simulink model "sgMdl_IO324_AnalogLoopbackDMA"  (R2024b)
settings: Solver=FixedStepAuto  StartTime=0.0  StopTime=inf  RelTol=1e-3
undefined symbols (not defined in the file): Ended, IO3xx, Pull, pull, Single, up
libraries: slrealtimeloglib x7, speedgoatlib_fpga_analog_io x3, speedgoatlib_interrupt x2, speedgoatlib_fpga x1
Description:
  | IO324 - Analog Loopback with DMA and Frame-Based Processing
settings Model: ModifiedByFormat=Speedgoat  SimulationMode=external  ExtModeTrigDuration=100000  Creator=Speedgoat  LastModifiedBy=Speedgoat
settings SolverCC: ConcurrentTasks=on  PositivePriorityOrder=on
settings DataIOCC: SaveFormat=StructureWithTime
settings OptimizationCC: BlockReduction=off  OptimizeBlockIOStorage=off  BufferReuse=off  ReuseModelBlockBuffer=off
settings DebuggingCC: UnderspecifiedInitializationDetection=Classic  MergeDetectMultiDrivingBlocksExec=none  TasksWithSamePriorityMsg=none
settings HardwareCC: ProdBitPerLong=64  ProdLongLongMode=on  ProdHWDeviceType=Intel->x86-64 (Linux 64)
settings ModelReferenceCC: EnableRefExpFcnMdlSchedulingChecks=on  PropagateSignalLabelsOutOfModel=off
settings RTWCC: Description=Speedgoat Real-Time Target Machine  SystemTargetFile=speedgoat.tlc  TemplateMakefile=slrealtime_default_tmf  PostCodeGenCommand=sg.model.build.makeCfg(bdroot, buildInfo);  Toolchain=Simulink Real-Time Toolchain  BuildConfiguration=Faster Runs  TargetLang=C++  GPUComputeCapability=3.5
settings SimulinkRealTimeTargetCC: SubcomponentCodeInterfacePackaging=Reusable function  InstructionSetFMA=off  LogToMDFFile=off  SLRTForcePollingMode=on  SLRTFileLogMaxRuns=10
settings ConfigComp: CovBoundaryAbsTol=1.0e-5

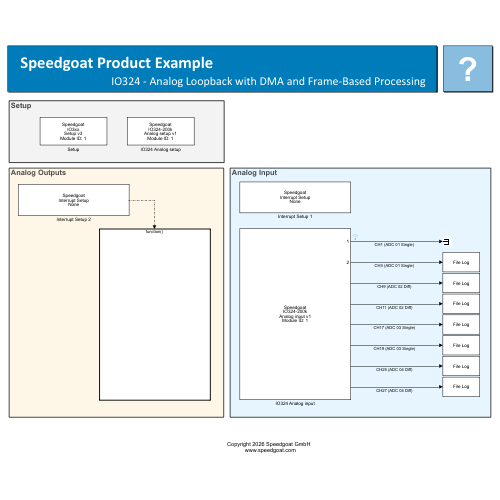
[thumbnail: Simulink's stored preview of the top-level diagram]
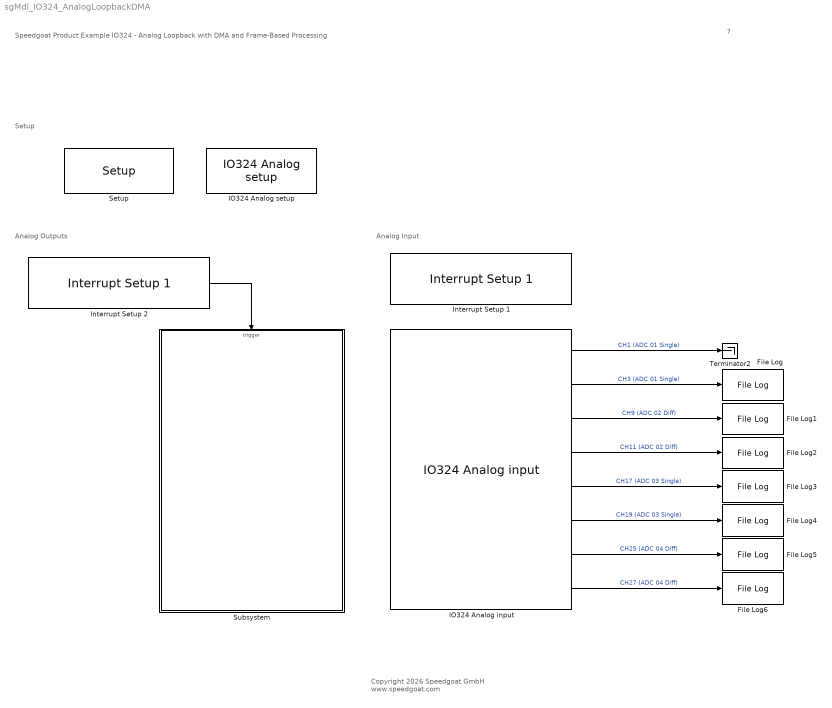
== system sgMdl_IO324_AnalogLoopbackDMA ==
  note: Analog Outputs
  note: Analog Input
  note: Setup
  note: Speedgoat Product Example
      | IO324 - Analog Loopback with DMA and Frame-Based Processing
  note: ?
  note: Copyright 2026 Speedgoat GmbH
      |  www.speedgoat.com
  File Log{,1..6} (7 alike) : slrealtimeloglib/File Log  decimation=1  inputProcessing=Elements as channels (sample based)
  IO324 Analog input : speedgoatlib_fpga_analog_io/IO324/IO324 Analog input  Priority=1  id=1  parSampleTime=-1  parPciSlot=-1  parAiChannels=[1 3 9 11 17 19 25 27]  parAiTriggerMode=[2 2 2 2]  parAiReadPrevValue=0  parAiEnableFrame=1  parAiVoltageRange=[2 2 2 2 2 2 2 2]  parAdcCoupling=[1 1 1 1]  parAdcContSampling=0  parAdcDmaEnable=0  parAdcActiveDmaDevices=[1 1 1 1]  parAiFrameSize=100
      settings: SourceProductName=Simulink Real-Time: Speedgoat I/O Blockset
  IO324 Analog setup : speedgoatlib_fpga_analog_io/IO324/IO324 Analog setup  id=1  parEnableCodeModule1=off  parEnableCodeModule2=off  parEnableCodeModule3=off  parEnableCodeModule4=off  parEnableCodeModule5=off  parEnableCodeModule6=off  parEnableCodeModule7=off  parEnableCodeModule8=off  parAdcEnableIndividualTrigger=off  parAdcTriggerMode1=Model Step  parAdcSampleRate1=100e3  parAdcDioTriggerChannel1=1  parAdcInternalTrigger1=<empty>  parAdcOversampling1=None  parAdcTriggerMode2=Model Step  parAdcSampleRate2=100e3  parAdcDioTriggerChannel2=1  parAdcInternalTrigger2=<empty>  parAdcOversampling2=None  parAdcTriggerMode3=Model Step  parAdcSampleRate3=100e3  parAdcDioTriggerChannel3=1  parAdcInternalTrigger3=<empty>  parAdcOversampling3=None  parAdcTriggerMode4=Model Step  parAdcSampleRate4=100e3  parAdcDioTriggerChannel4=1  parAdcInternalTrigger4=<empty>  parAdcOversampling4=None  parAdcReadPrevValueIndividualTrigger=on  parAdcEnableFrame=on  parAdcTriggerMode=I/O Module Clock  parAdcReadPrevValue=off  parAdcSampleRate=100e3  parAdcDioTriggerChannel=1  parAdcInternalTrigger=<empty>  parAdcOversampling=None  parAdcTriggerResolution=1e-08  parAdcSampleRateFrame=250e3  parAdcFrameSize=100  parAdcSampleTime=-1  parDacTriggerMode=I/O Module Clock  parDacInternalTrigger=<empty>  parDacDioTriggerChannel=0  parDacEnableFrame=on  dacUsesTimer=off  parDacFifoThreshold=25  parDacTriggerResolution=1e-08  parDacSampleRate=250e3  parDacFrameSize=1000  parDacSampleTime=-1  parAdcCoupling1=Single-Ended  parAdcChannel1=on  parAdcChannel2=off  parAdcChannel3=on  parAdcChannel4=off  parAdcChannel5=off  parAdcChannel6=off  parAdcChannel7=off  parAdcChannel8=off  parAdcRangeAll1=+-10.24 V  parVoltageRangePerChannelEn1=off  parAdcRange1=+-10.24 V  parAdcRange5=+-10.24 V  parAdcRange2=+-10.24 V  parAdcRange6=+-10.24 V  parAdcRange3=+-10.24 V  parAdcRange7=+-10.24 V  parAdcRange4=+-10.24 V  parAdcRange8=+-10.24 V  parAdcCoupling2=Differential  parAdcChannel9=on  parAdcChannel10=on  parAdcChannel11=on  parAdcChannel12=off  parAdcChannel13=off  parAdcChannel14=off  parAdcChannel15=off  parAdcChannel16=off  parAdcRangeAll2=+-10.24 V  parVoltageRangePerChannelEn2=off  parAdcRange9=+-10.24 V  parAdcRange13=+-10.24 V  parAdcRange10=+-10.24 V  parAdcRange14=+-10.24 V  parAdcRange11=+-10.24 V  parAdcRange15=+-10.24 V  parAdcRange12=+-10.24 V  parAdcRange16=+-10.24 V  parAdcCoupling3=Single-Ended  parAdcChannel17=on  parAdcChannel18=off  parAdcChannel19=on  parAdcChannel20=off  parAdcChannel21=off  parAdcChannel22=off  parAdcChannel23=off  parAdcChannel24=off  parAdcRangeAll3=+-10.24 V  parVoltageRangePerChannelEn3=off  parAdcRange17=+-10.24 V  parAdcRange21=+-10.24 V  parAdcRange18=+-10.24 V  parAdcRange22=+-10.24 V  parAdcRange19=+-10.24 V  parAdcRange23=+-10.24 V  parAdcRange20=+-10.24 V  parAdcRange24=+-10.24 V  parAdcCoupling4=Differential  parAdcChannel25=on  parAdcChannel26=on  parAdcChannel27=on  parAdcChannel28=off  parAdcChannel29=off  parAdcChannel30=off  parAdcChannel31=off  parAdcChannel32=off  parAdcRangeAll4=+-10.24 V  parVoltageRangePerChannelEn4=off  parAdcRange25=+-10.24 V  parAdcRange29=+-10.24 V  parAdcRange26=+-10.24 V  parAdcRange30=+-10.24 V  parAdcRange27=+-10.24 V  parAdcRange31=+-10.24 V  parAdcRange28=+-10.24 V  parAdcRange32=+-10.24 V  parAdcAutoCorrection=on  parDacChannel1=on  parDacChannel2=on  parDacChannel3=on  parDacChannel4=on  parDacChannel5=on  parDacChannel6=on  parDacChannel7=on  parDacChannel8=on  parDacRange1=+-10 V  parDacInitValue1=-10  parDacReset1=on  parDacRange2=+-10 V  parDacInitValue2=-9  parDacReset2=off  parDacRange3=+-10 V  parDacInitValue3=-8  parDacReset3=on  parDacRange4=+-10 V  parDacInitValue4=-7  parDacReset4=off  parDacRange5=+-10 V  parDacInitValue5=-6  parDacReset5=on  parDacRange6=+-10 V  parDacInitValue6=-5  parDacReset6=off  parDacRange7=+-10 V  parDacInitValue7=-4  parDacReset7=on  parDacRange8=+-10 V  parDacInitValue8=-3  parDacReset8=off  parDacAutoCorrection=on
      settings: SourceProductName=Simulink Real-Time: Speedgoat I/O Blockset
  Interrupt Setup 1 : speedgoatlib_interrupt/Interrupt Setup 1  parModuleTrigger=on  parPollingMode=off  parPriorityConf=High  parPriority=241  confStartFcn=IO324_200k_ANALOG_IN_start_public  confStopFcn=IO324_200k_ANALOG_IN_stop_public  confIsrFcn=IO324_200k_ANALOG_IN_isr_public  confMapFcn=IO324_200k_ANALOG_IN_map_public  confHookFile=io324_200k_analog_in_int_hooks.c  confIrqNr=-1  confIsPolling=off  confModID=16776961  confSelectedInt=Speedgoat IO324-200k Analog input interrupt  confSelectedId=1  confSelectedChannel=[]  confData=[90 1]  confForcePollingMode=off
  Interrupt Setup 2 : speedgoatlib_interrupt/Interrupt Setup 1  parModuleTrigger=off  parPollingMode=off  parPriorityConf=High  parPriority=241  confStartFcn=IO324_200k_ANALOG_OUT_start_public  confStopFcn=IO324_200k_ANALOG_OUT_stop_public  confIsrFcn=IO324_200k_ANALOG_OUT_isr_public  confMapFcn=IO324_200k_ANALOG_OUT_map_public  confHookFile=io324_200k_analog_out_int_hooks.c  confIrqNr=-1  confIsPolling=off  confModID=16776961  confSelectedInt=Speedgoat IO324-200k Analog output interrupt  confSelectedId=1  confSelectedChannel=[]  confData=[254 0]  confForcePollingMode=off
  Setup : speedgoatlib_fpga/Setup/Setup  board=Please select...  id=1  pciSlot=-1  device_id=1  bitstreamFilePath=[]  bitstreamFile=Please select...  fpgaFreq=[100000000 100000000]  enableDma=on  rearEnb_1=off  rearIO_1=IO3xx-21  rearEnb_2=off  rearIO_2=None  ProgSpiFlash=off  ProgBPIFlash=off  useFpgaDmaController=off  dmaTrigDropdown=Model Step  dmaTrigSelect=0  dmaStopOnOverload=on  dmaModeSequential=on  dmaModeParallel=off  PullRPort15=pull-up 3.3V  PullRPort31=pull-up 3.3V  PullRPort47=pull-up 3.3V  PullRPort63=pull-up 3.3V  diffLineTermination_1=on  diffLineTermination_2=on  diffLineTermination_3=on  diffLineTermination_4=on  diffLineTermination_5=on  diffLineTermination_6=on  diffLineTermination_7=on  diffLineTermination_8=on  diffLineTermination_9=on  diffLineTermination_10=on  diffLineTermination_11=on  diffLineTermination_12=on  diffLineTermination_13=on  diffLineTermination_14=on  diffLineTermination_15=on  diffLineTermination_16=on  diffLineTermination_17=on  diffLineTermination_18=on  diffLineTermination_19=on  diffLineTermination_20=on  diffLineTermination_21=on  diffLineTermination_22=on  diffLineTermination_23=on  diffLineTermination_24=on  diffLineTermination_25=on  diffLineTermination_26=on  diffLineTermination_27=on  diffLineTermination_28=on  diffLineTermination_29=on  diffLineTermination_30=on  diffLineTermination_31=on  diffLineTermination_32=on  ioVoltageDropDown1=3.3V  pullResistorDropDown1_1=Pull-up  pullResistorDropDown1_2=Pull-up  pullResistorDropDown1_3=Pull-up  pullResistorDropDown1_4=Pull-up  pullResistorDropDown1_5=Pull-up  pullResistorDropDown1_6=Pull-up  pullResistorDropDown1_7=Pull-up  pullResistorDropDown1_8=Pull-up  ttlIsImplementedCheckBox1=off  pullResistorDropDown2=Pull-up  ioVoltageDropDown2=3.3V  ttlIsImplementedCheckBox2=off  pullResistorDropDown3=Pull-up  ioVoltageDropDown3=3.3V  ttlIsImplementedCheckBox3=off  pullResistorDropDown4=Pull-up  ioVoltageDropDown4=3.3V  ttlIsImplementedCheckBox4=off  pullResistorDropDown5=Pull-up  ioVoltageDropDown5=3.3V  ttlIsImplementedCheckBox5=off  pullResistorDropDown6=Pull-up  ioVoltageDropDown6=3.3V  ttlIsImplementedCheckBox6=off  pullResistorDropDown7=Pull-up  ioVoltageDropDown7=3.3V  ttlIsImplementedCheckBox7=off  pullResistorDropDown8=Pull-up  ioVoltageDropDown8=3.3V  ttlIsImplementedCheckBox8=off  terminationCheckBox1=off  terminationCheckBox2=off  terminationCheckBox3=off  terminationCheckBox4=off  diffIsImplementedCheckBox1=off  terminationCheckBox5=off  terminationCheckBox6=off  terminationCheckBox7=off  terminationCheckBox8=off  diffIsImplementedCheckBox2=off  terminationCheckBox9=off  terminationCheckBox10=off  terminationCheckBox11=off  terminationCheckBox12=off  diffIsImplementedCheckBox3=off  terminationCheckBox13=off  terminationCheckBox14=off  terminationCheckBox15=off  terminationCheckBox16=off  diffIsImplementedCheckBox4=off  terminationCheckBox17=off  terminationCheckBox18=off  terminationCheckBox19=off  terminationCheckBox20=off  diffIsImplementedCheckBox5=off  terminationCheckBox21=off  terminationCheckBox22=off  terminationCheckBox23=off  terminationCheckBox24=off  diffIsImplementedCheckBox6=off  terminationCheckBox25=off  terminationCheckBox26=off  terminationCheckBox27=off  terminationCheckBox28=off  diffIsImplementedCheckBox7=off  terminationCheckBox29=off  terminationCheckBox30=off  terminationCheckBox31=off  terminationCheckBox32=off  diffIsImplementedCheckBox8=off  PullRPort0_1=pull-up  VioPort0_1=3.3V  PullRPort1_1=pull-up  VioPort1_1=3.3V  PullRPort2_1=pull-up  VioPort2_1=3.3V  PullRPort3_1=pull-up  VioPort3_1=3.3V  PullRPort4_1=pull-up  VioPort4_1=3.3V  PullRPort5_1=pull-up  VioPort5_1=3.3V  PullRPort6_1=pull-up  VioPort6_1=3.3V  diffLineTermination_rear1_1=on  diffLineTermination_rear1_2=on  diffLineTermination_rear1_3=on  diffLineTermination_rear1_4=on  diffLineTermination_rear1_5=on  diffLineTermination_rear1_6=on  diffLineTermination_rear1_7=on  diffLineTermination_rear1_8=on  PullRPort0_2=pull-up  VioPort0_2=3.3V  PullRPort1_2=pull-up  VioPort1_2=3.3V  PullRPort2_2=pull-up  VioPort2_2=3.3V  PullRPort3_2=pull-up  VioPort3_2=3.3V  PullRPort4_2=pull-up  VioPort4_2=3.3V  PullRPort5_2=pull-up  VioPort5_2=3.3V  PullRPort6_2=pull-up  VioPort6_2=3.3V  diffLineTermination_rear2_1=on  diffLineTermination_rear2_2=on  diffLineTermination_rear2_3=on  diffLineTermination_rear2_4=on  diffLineTermination_rear2_5=on  diffLineTermination_rear2_6=on  diffLineTermination_rear2_7=on  diffLineTermination_rear2_8=on
      settings: SourceProductName=IO3xx
  Subsystem : Subsystem
  Terminator2 : Terminator
  wires:
  Interrupt Setup 2/1 -> Subsystem/Trigger
  IO324 Analog input/5 -> File Log3/1  "CH17 (ADC 03 Single)"
  IO324 Analog input/3 -> File Log1/1  "CH9 (ADC 02 Diff)"
  IO324 Analog input/8 -> File Log6/1  "CH27 (ADC 04 Diff)"
  IO324 Analog input/2 -> File Log/1  "CH3 (ADC 01 Single)"
  IO324 Analog input/6 -> File Log4/1  "CH19 (ADC 03 Single)"
  IO324 Analog input/1 -> Terminator2/1  "CH1 (ADC 01 Single)"
  IO324 Analog input/7 -> File Log5/1  "CH25 (ADC 04 Diff)"
  IO324 Analog input/4 -> File Log2/1  "CH11 (ADC 02 Diff)"

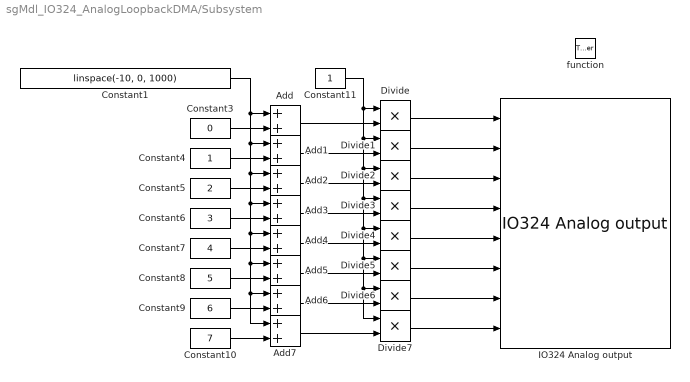
== system sgMdl_IO324_AnalogLoopbackDMA/Subsystem ==
  function : TriggerPort  TriggerType=function-call  VariantControl=(inherit)
  Add{,1..7} (8 alike) : Sum
  Constant1 : Constant  Value=linspace(-10, 0, 1000)  SampleTime=-1
  Constant10 : Constant  Value=7  SampleTime=-1
  Constant11 : Constant  SampleTime=-1
  Constant3 : Constant  Value=0  SampleTime=-1
  Constant4 : Constant  SampleTime=-1
  Constant5 : Constant  Value=2  SampleTime=-1
  Constant6 : Constant  Value=3  SampleTime=-1
  Constant7 : Constant  Value=4  SampleTime=-1
  Constant8 : Constant  Value=5  SampleTime=-1
  Constant9 : Constant  Value=6  SampleTime=-1
  Divide{,1..7} (8 alike) : Product  Inputs=**
  IO324 Analog output : speedgoatlib_fpga_analog_io/IO324/IO324 Analog output  Priority=2  id=1  parSampleTime=-1  parPciSlot=-1  parAoChannels=[1 2 3 4 5 6 7 8]  parAoVoltageRange=[1 1 1 1 1 1 1 1]  parDacOverRange=[0 0 0 0 0 0 0 0]  parAoInitValues=[-10 -9 -8 -7 -6 -5 -4 -3]  parAoReset=[1 0 1 0 1 0 1 0]  parDacSyncOut=1  parAoEnableFrame=1  parDacActiveDmaDevices=[1 1 1 1]  parDacDmaLatency=2  parAoFrameSize=1000
      settings: SourceProductName=Simulink Real-Time: Speedgoat I/O Blockset
  wires:
  Constant1/1 -> Add7/1, Add6/1, Add5/1, Add4/1, Add3/1, Add2/1, Add1/1, Add/1
  Constant3/1 -> Add/2
  Constant4/1 -> Add1/2
  Constant5/1 -> Add2/2
  Constant6/1 -> Add3/2
  Constant7/1 -> Add4/2
  Constant8/1 -> Add5/2
  Constant9/1 -> Add6/2
  Constant10/1 -> Add7/2
  Add/1 -> Divide/2
  Add1/1 -> Divide1/2
  Add2/1 -> Divide2/2
  Add3/1 -> Divide3/2
  Add4/1 -> Divide4/2
  Add5/1 -> Divide5/2
  Add6/1 -> Divide6/2
  Add7/1 -> Divide7/2
  Constant11/1 -> Divide7/1, Divide6/1, Divide5/1, Divide4/1, Divide3/1, Divide2/1, Divide1/1, Divide/1
  Divide/1 -> IO324 Analog output/1
  Divide1/1 -> IO324 Analog output/2
  Divide2/1 -> IO324 Analog output/3
  Divide3/1 -> IO324 Analog output/4
  Divide4/1 -> IO324 Analog output/5
  Divide5/1 -> IO324 Analog output/6
  Divide6/1 -> IO324 Analog output/7
  Divide7/1 -> IO324 Analog output/8
